simulink model "MotoSimpleEngine"  (R2026b)
settings: Solver=VariableStepAuto
libraries: autolibsharedcommon x1, autolibsharedmappedengines x1
settings Model: ModifiedByFormat=The MathWorks, Inc.  Creator=The MathWorks, Inc.  LastModifiedBy=The MathWorks, Inc.

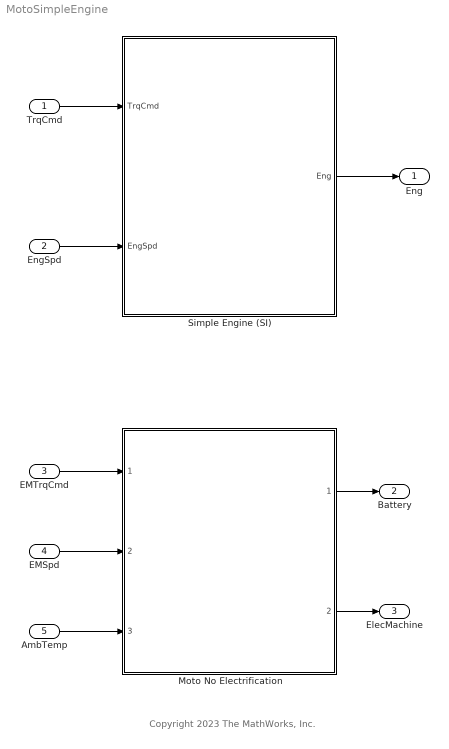
== system MotoSimpleEngine ==
  note: Copyright 2023 The MathWorks, Inc.
  TrqCmd : Inport
  EngSpd : Inport  Port=2
  EMTrqCmd : Inport  Port=3
  EMSpd : Inport  Port=4
  AmbTemp : Inport  Port=5
  Moto No Electrification : Subsystem  VariantControl=Moto No Electrification  ReferencedSubsystem=NoElectrical
  Simple Engine (SI) : Subsystem  VariantControl=Simple Engine (SI)
  Eng : Outport
  Battery : Outport  Port=2
  ElecMachine : Outport  Port=3
  wires:
  TrqCmd/1 -> Simple Engine (SI)/1(TrqCmd)
  EngSpd/1 -> Simple Engine (SI)/2(EngSpd)
  Simple Engine (SI)/1(Eng) -> Eng/1
  AmbTemp/1 -> Moto No Electrification/3
  EMSpd/1 -> Moto No Electrification/2
  EMTrqCmd/1 -> Moto No Electrification/1
  Moto No Electrification/2 -> ElecMachine/1
  Moto No Electrification/1 -> Battery/1

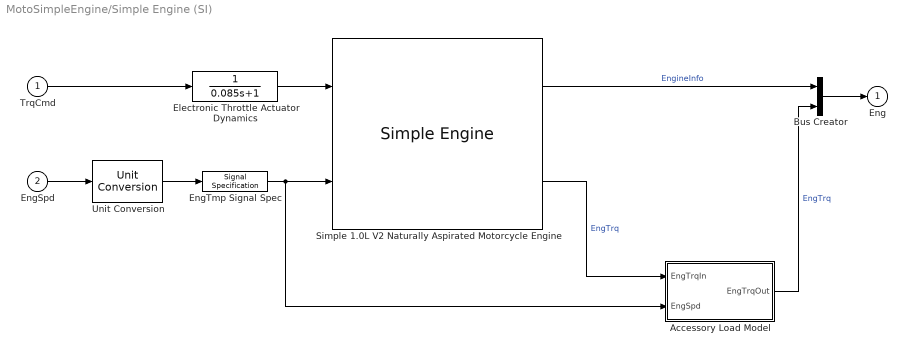
== system MotoSimpleEngine/Simple Engine (SI) ==
  TrqCmd : Inport
  EngSpd : Inport  Port=2
  Accessory Load Model : Subsystem
  Bus Creator : BusCreator  Inputs=2
  Electronic Throttle Actuator Dynamics : TransferFcn  Denominator=[0.085 1]
  EngTmp Signal Spec : SignalSpecification  Unit=rpm
  Simple 1.0L V2 Naturally Aspirated Motorcycle Engine : autolibsharedmappedengines/Simple Engine  f_tqmax=PlntEngTqMax  f_tqmax_n_bpt=PlntEngTqMaxBpt  Lhv=PlntEngLhv  Sg=PlntEngSg  BsfcAvg=PlntEngBsfcAvg  aMode=2
      settings: LibrarySourceBlock=vdynlib/Powertrain/Propulsion/Simple Engine
  Unit Conversion : UnitConversion
  Eng : Outport
  wires:
  Accessory Load Model/1(EngTrqOut) -> Bus Creator/2  "EngTrq"
  Bus Creator/1 -> Eng/1
  Electronic Throttle Actuator Dynamics/1 -> Simple 1.0L V2 Naturally Aspirated Motorcycle Engine/1
  Simple 1.0L V2 Naturally Aspirated Motorcycle Engine/2 -> Accessory Load Model/1(EngTrqIn)  "EngTrq"
  Unit Conversion/1 -> EngTmp Signal Spec/1
  EngTmp Signal Spec/1 -> Accessory Load Model/2(EngSpd), Simple 1.0L V2 Naturally Aspirated Motorcycle Engine/2
  Simple 1.0L V2 Naturally Aspirated Motorcycle Engine/1 -> Bus Creator/1  "EngineInfo"
  TrqCmd/1 -> Electronic Throttle Actuator Dynamics/1
  EngSpd/1 -> Unit Conversion/1

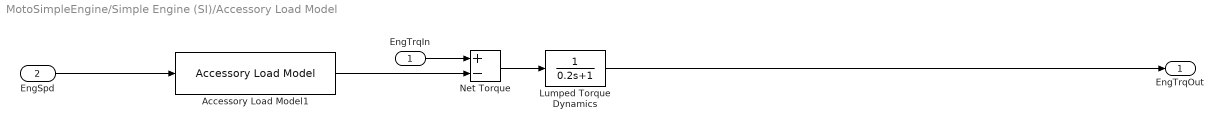
== system MotoSimpleEngine/Simple Engine (SI)/Accessory Load Model ==
  EngTrqIn : Inport
  EngSpd : Inport  Port=2
  Accessory Load Model1 : autolibsharedcommon/Accessory Load Model  AccPwrTbl=PlntEngAccPwrTbl  AccSpdBpts=PlntEngAccSpdBpt  aMode=aMode
  Lumped Torque Dynamics : TransferFcn  Denominator=[0.2 1]
  Net Torque : Sum  Inputs=+-
  EngTrqOut : Outport  Unit=N*m  VectorParamsAs1DForOutWhenUnconnected=off
  wires:
  Net Torque/1 -> Lumped Torque Dynamics/1
  Lumped Torque Dynamics/1 -> EngTrqOut/1
  Accessory Load Model1/1 -> Net Torque/2
  EngSpd/1 -> Accessory Load Model1/1
  EngTrqIn/1 -> Net Torque/1
